simulink model "test2"  (R2014b)
settings: Solver=ode45  StartTime=0.0  StopTime=inf  RelTol=1e-3
InitFcn:
  | mpsk = 4;
  | Fs = 915000000;
libraries: simulink x2, commdigbbndpm3 x1, siglabs_lib x1, commrandsrc2 x1
settings Model: Creator=Ben  LastModifiedBy=Ben

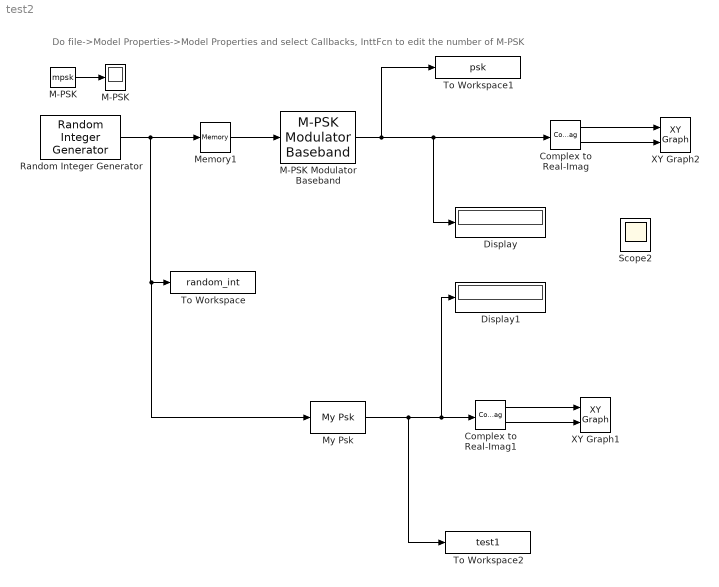
== system test2 ==
  note: Do file->Model Properties->Model Properties and select Callbacks, InttFcn to edit the number of M-PSK
  Complex to Real-Imag : ComplexToRealImag
  Complex to Real-Imag1 : ComplexToRealImag
  Display : Display
  Display1 : Display
  M-PSK : Display
  "M-PSK " : Constant  Value=mpsk
  M-PSK Modulator Baseband : commdigbbndpm3/M-PSK Modulator Baseband  M=mpsk  InType=Integer  Enc=Binary  Mapping=[0:7]  Ph=pi/4  outDtype=double  outWordLen=16  outUDDataType=sfix(16)  outFracLenMode=Best precision  outFracLen=15
  Memory1 : Memory  InheritSampleTime=on  LinearizeMemory=on
  My Psk : siglabs_lib/My Psk  SampsPerSym=8
  Random Integer Generator : commrandsrc2/Random Integer Generator  mul=mpsk  seed=43  Ts=.1  frameBased=off  sampPerFrame=1  orient=off  outDataType=double
  Scope2 : Scope  NumInputPorts=2
      settings: YMin=-5~-5  YMax=5~5
  To Workspace : ToWorkspace  VariableName=random_int  SampleTime=-1
      settings: Save2DSignal=2-D array (concatenate along first dimension)
  To Workspace1 : ToWorkspace  VariableName=psk  SampleTime=-1
      settings: Save2DSignal=2-D array (concatenate along first dimension)
  To Workspace2 : ToWorkspace  VariableName=test1  SampleTime=-1
      settings: Save2DSignal=2-D array (concatenate along first dimension)
  XY Graph1 : simulink/Sinks/XY Graph  xmin=-1  xmax=1  ymin=-1  ymax=1  st=-1
  XY Graph2 : simulink/Sinks/XY Graph  xmin=-1  xmax=1  ymin=-1  ymax=1  st=-1
  wires:
  Complex to Real-Imag/1 -> XY Graph2/1
  Complex to Real-Imag/2 -> XY Graph2/2
  "M-PSK "/1 -> M-PSK/1
  Complex to Real-Imag1/2 -> XY Graph1/2
  Complex to Real-Imag1/1 -> XY Graph1/1
  My Psk/1 -> To Workspace2/1, Display1/1, Complex to Real-Imag1/1
  M-PSK Modulator Baseband/1 -> Display/1, Complex to Real-Imag/1, To Workspace1/1
  Random Integer Generator/1 -> Memory1/1, My Psk/1, To Workspace/1
  Memory1/1 -> M-PSK Modulator Baseband/1
